simulink model "aliasing_demo"  (R2023a)
settings: Solver=ode45  StartTime=0.0  StopTime=1  RelTol=1e-3  EnableMultiTasking=on
settings Model: Creator=rcheng  LastModifiedBy=ribei
settings SolverCC: AlgebraicLoopSolver=TrustRegion
settings DataIOCC: LimitDataPoints=on  SaveFormat=Array  SignalLoggingSaveFormat=ModelDataLogs  ReturnWorkspaceOutputs=off
settings OptimizationCC: ExpressionDepthLimit=2147483647  InitFltsAndDblsToZero=on  LifeSpan=inf
settings DebuggingCC: UnderspecifiedInitializationDetection=Classic  MergeDetectMultiDrivingBlocksExec=none  SolverPrmCheckMsg=warning  FcnCallInpInsideContextMsg=warning  UnconnectedInputMsg=warning  UnconnectedOutputMsg=warning  UnconnectedLineMsg=warning  StateNameClashWarn=warning  SFUnexpectedBacktrackingDiag=warning  SFNoUnconditionalDefaultTransitionDiag=warning  SFExecutionAtInitializationDiag=none  ArithmeticOperatorsInVariantConditions=warning
settings HardwareCC: ProdBitPerPointer=32  ProdBitPerSizeT=32  ProdBitPerPtrDiffT=32  ProdLargestAtomicFloat=None  ProdIntDivRoundTo=Undefined  ProdEndianess=Unspecified  ProdWordSize=32  ProdHWDeviceType=32-bit Generic
settings ModelReferenceCC: EnableRefExpFcnMdlSchedulingChecks=on  PropagateSignalLabelsOutOfModel=off
settings SFSimCC: SimUseLocalCustomCode=off  CustomCodeUndefinedFunction=UseInterfaceOnly
settings RTWCC: RTWUseLocalCustomCode=off
settings CodeAppCC: StateflowObjectComments=on
settings GRTTargetCC: TargetLangStandard=C89/C90 (ANSI)  CombineOutputUpdateFcns=off  GRTInterface=on
settings ConfigComp: CovMetricSettings=dw  CovSaveCumulativeToWorkspaceVar=on  CovSaveSingleToWorkspaceVar=on  CovExternalEMLEnable=off  CovSFcnEnable=off

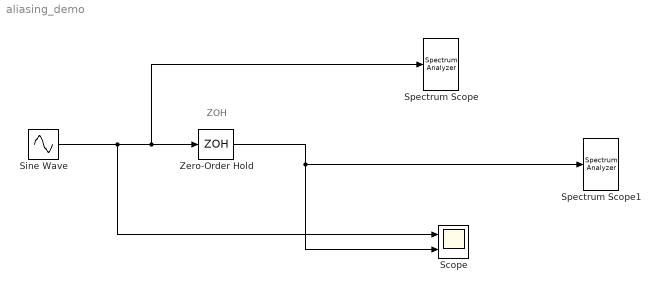
== system aliasing_demo ==
  note: ZOH
  Scope : Scope  NumInputPorts=2
  Sine Wave : Sin  Amplitude=5  Frequency=2*pi*100  SampleTime=1/10000
  Spectrum Scope : SpectrumAnalyzer  WindowPosition=[62.000000,294.000000,955.000000,580.000000,]  ScopeFrameLocation=window  Method=Welch  PlotAsTwoSidedSpectrum=off  AxesScaling=Manual  Span=37.5  CenterFrequency=18.75  StartFrequency=0  StopFrequency=37.5  FrequencyResolutionMethod=Window length  FFTLength=128  WindowLength=128  OverlapPercent=50  AveragingMethod=Running  SpectralAverages=2  SpectrumUnits=dBW  YLabel=Magnitude-squared  YLimits=[-37.971666823755732878,14.06500178037488169]  DefaultConfigurationName=spbscopes.SpectrumAnalyzerBlockCfg  IsFrequencyInputMode=0  FrequencyVectorPort=0  FrequencyVectorFromPort=0  FrequencyInputRBWPort=0  FrequencyInputRBWFromPort=0
  Spectrum Scope1 : SpectrumAnalyzer  WindowPosition=[601.000000,291.000000,955.000000,580.000000,]  ScopeFrameLocation=window  Method=Welch  PlotAsTwoSidedSpectrum=off  AxesScaling=Manual  Span=37.5  CenterFrequency=18.75  StartFrequency=0  StopFrequency=37.5  FrequencyResolutionMethod=Window length  FFTLength=128  WindowLength=128  OverlapPercent=50  AveragingMethod=Running  SpectralAverages=2  SpectrumUnits=dBW  YLabel=Magnitude-squared  YLimits=[-37.971666823755732878,14.06500178037488169]  DefaultConfigurationName=spbscopes.SpectrumAnalyzerBlockCfg  IsFrequencyInputMode=0  FrequencyVectorPort=0  FrequencyVectorFromPort=0  FrequencyInputRBWPort=0  FrequencyInputRBWFromPort=0
  Zero-Order Hold : ZeroOrderHold  SampleTime=1/1000
  wires:
  Zero-Order Hold/1 -> Scope/2, Spectrum Scope1/1
  Sine Wave/1 -> Scope/1, Spectrum Scope/1, Zero-Order Hold/1
